simulink model "sampleModel2072_pp"  (R2021a)
settings: Solver=VariableStepAuto  StartTime=0.0  StopTime=10.0  RelTol=1e-3
undefined symbols (not defined in the file or in its folder): DiscIntNeverNeededParam, magnitude, Newton, Raphson
libraries: simulink x184, pid_lib x33
(part 1 of 5)
settings Model: Creator=user  LastModifiedBy=user

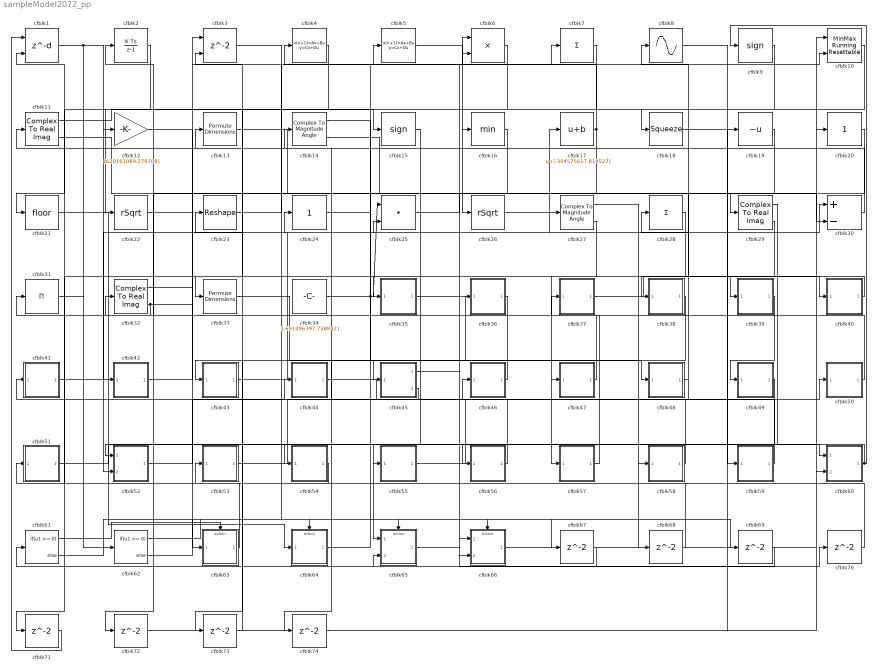
== system sampleModel2072_pp ==
  cfblk1 : Delay  DelayLengthSource=Input port  SampleTime=1
      settings: InputPortMap=u0,p1
  cfblk10 : simulink/Math Operations/MinMax Running Resettable  Function=min  vinit=0.0
  cfblk11 : ComplexToRealImag
  cfblk12 : Gain  Gain=[620161089.279708]
  cfblk13 : PermuteDimensions
  cfblk14 : ComplexToMagnitudeAngle
  cfblk15 : Signum
  cfblk16 : MinMax
  cfblk17 : Bias  Bias=[-304575617.814527]
  cfblk18 : Squeeze
  cfblk19 : UnaryMinus
  cfblk2 : DiscreteIntegrator  ICPrevOutput=DiscIntNeverNeededParam  ICPrevScaledInput=DiscIntNeverNeededParam
  cfblk20 : simulink/Math Operations/Slider Gain  gain=1  low=0  high=2
  cfblk21 : Rounding
  cfblk22 : Sqrt  Operator=rSqrt  AlgorithmType=Newton-Raphson  SaturateOnIntegerOverflow=on
  cfblk23 : Reshape
  cfblk24 : simulink/Math Operations/Slider Gain  gain=1  low=0  high=2
  cfblk25 : DotProduct  InputSameDT=on  OutDataTypeStr=Inherit: Inherit via internal rule
  cfblk26 : Sqrt  Operator=rSqrt  AlgorithmType=Newton-Raphson  SaturateOnIntegerOverflow=on
  cfblk27 : ComplexToMagnitudeAngle
  cfblk28 : Sum  Inputs=+
  cfblk29 : ComplexToRealImag
  cfblk3 : Delay  ShowEnablePort=on  SampleTime=1
      settings: InputPortMap=u0,e6
  cfblk30 : Sum  Inputs=+-
  cfblk31 : Product  Inputs=*
  cfblk32 : ComplexToRealImag
  cfblk33 : PermuteDimensions
  cfblk34 : Constant  Value=[-691496397.738842]  SampleTime=1
  cfblk35 : Subsystem
  cfblk36 : Subsystem
  cfblk37 : Subsystem
  cfblk38 : Subsystem
  cfblk39 : Subsystem
  cfblk4 : DiscreteStateSpace
  cfblk40 : Subsystem
  cfblk41 : Subsystem
  cfblk42 : Subsystem
  cfblk43 : Subsystem
  cfblk44 : Subsystem
  cfblk45 : Subsystem
  cfblk46 : Subsystem
  cfblk47 : Subsystem
  cfblk48 : Subsystem
  cfblk49 : Subsystem
  cfblk5 : DiscreteStateSpace
  cfblk50 : Subsystem
  cfblk51 : Subsystem
  cfblk52 : Subsystem
  cfblk53 : Subsystem
  cfblk54 : Subsystem
  cfblk55 : Subsystem
  cfblk56 : Subsystem
  cfblk57 : Subsystem
  cfblk58 : Subsystem
  cfblk59 : Subsystem
  cfblk6 : Product  Inputs=**
  cfblk60 : Subsystem
  cfblk61 : If  IfExpression=u1 >= 0  SampleTime=1
  cfblk62 : If  IfExpression=u1 >= 0  SampleTime=1
  cfblk63 : Subsystem  TreatAsAtomicUnit=on
  cfblk64 : Subsystem  TreatAsAtomicUnit=on
  cfblk65 : Subsystem  TreatAsAtomicUnit=on
  cfblk66 : Subsystem  TreatAsAtomicUnit=on
  cfblk{67..74} (8 alike) : Delay  SampleTime=1
  cfblk7 : Sum  Inputs=+
  cfblk8 : Sin  TimeSource=Use external signal  SampleTime=0
  cfblk9 : Signum
  wires:
  cfblk10/1 -> cfblk18/1
  cfblk51/1(cfblk2) -> cfblk60/1(cfblk1)
  cfblk35/1(cfblk2) -> cfblk48/1(cfblk1)
  cfblk21/1 -> cfblk64/1(cfblk1)
  cfblk54/1(cfblk2) -> cfblk53/1(cfblk1)
  cfblk34/1 -> cfblk25/1, cfblk7/1
  cfblk4/1 -> cfblk33/1
  cfblk26/1 -> cfblk27/1
  cfblk60/1(cfblk2) -> cfblk9/1, cfblk56/1(cfblk1)
  cfblk39/1(cfblk2) -> cfblk49/1(cfblk1)
  cfblk8/1 -> cfblk59/1(cfblk1)
  cfblk2/1 -> cfblk22/1
  cfblk31/1 -> cfblk42/1(cfblk1)
  cfblk44/1(cfblk2) -> cfblk28/1
  cfblk56/1(cfblk2) -> cfblk23/1
  cfblk66/1(cfblk2) -> cfblk20/1
  cfblk29/1 -> cfblk52/1(cfblk1)
  cfblk30/1 -> cfblk11/1
  cfblk53/1(cfblk2) -> cfblk50/1(cfblk1)
  cfblk50/1(cfblk2) -> cfblk2/1
  cfblk24/1 -> cfblk6/1
  cfblk15/1 -> cfblk35/1(cfblk1)
  cfblk47/1(cfblk2) -> cfblk32/1
  cfblk49/1(cfblk2) -> cfblk65/1(cfblk1)
  cfblk40/1(cfblk2) -> cfblk39/1(cfblk1)
  cfblk9/1 -> cfblk26/1
  cfblk29/2 -> cfblk57/1(cfblk1)
  cfblk41/1(cfblk2) -> cfblk24/1
  cfblk59/1(cfblk2) -> cfblk46/1(cfblk1)
  cfblk46/1(cfblk2) -> cfblk43/1(cfblk1)
  cfblk32/1 -> cfblk3/1
  cfblk5/1 -> cfblk16/1
  cfblk48/1(cfblk2) -> cfblk8/1
  cfblk32/2 -> cfblk25/2, cfblk31/1
  cfblk13/1 -> cfblk36/1(cfblk1)
  cfblk43/1(cfblk2) -> cfblk17/1
  cfblk1/1 -> cfblk12/1, cfblk62/1
  cfblk64/1(cfblk2) -> cfblk30/1
  cfblk7/1 -> cfblk21/1
  cfblk37/1(cfblk2) -> cfblk40/1(cfblk1)
  cfblk19/1 -> cfblk38/1(cfblk1)
  cfblk23/1 -> cfblk5/1
  cfblk17/1 -> cfblk4/1, cfblk66/2(cfblk13)
  cfblk42/1(cfblk2) -> cfblk6/2
  cfblk20/1 -> cfblk45/1(cfblk1)
  cfblk55/1(cfblk2) -> cfblk10/1
  cfblk25/1 -> cfblk10/2
  cfblk11/1 -> cfblk15/1
  cfblk14/1 -> cfblk47/1(cfblk1)
  cfblk58/1(cfblk2) -> cfblk14/1
  cfblk14/2 -> cfblk29/1
  cfblk18/1 -> cfblk30/2
  cfblk6/1 -> cfblk52/2(cfblk16)
  cfblk52/1(cfblk2) -> cfblk44/1(cfblk1)
  cfblk12/1 -> cfblk54/1(cfblk1)
  cfblk57/1(cfblk2) -> cfblk37/1(cfblk1)
  cfblk22/1 -> cfblk63/1(cfblk1)
  cfblk11/2 -> cfblk66/1(cfblk1)
  cfblk27/1 -> cfblk58/1(cfblk1)
  cfblk63/1(cfblk2) -> cfblk51/1(cfblk1)
  cfblk27/2 -> cfblk55/1(cfblk1)
  cfblk45/2(cfblk14) -> cfblk41/1(cfblk1)
  cfblk61/1 -> cfblk63/Action
  cfblk61/2 -> cfblk64/Action
  cfblk62/1 -> cfblk65/Action
  cfblk62/2 -> cfblk66/Action
  cfblk3/1 -> cfblk67/1
  cfblk67/1 -> cfblk61/1
  cfblk33/1 -> cfblk68/1
  cfblk68/1 -> cfblk3/2
  cfblk45/1(cfblk2) -> cfblk69/1
  cfblk69/1 -> cfblk65/2(cfblk9)
  cfblk65/1(cfblk2) -> cfblk70/1
  cfblk70/1 -> cfblk1/2
  cfblk28/1 -> cfblk71/1
  cfblk71/1 -> cfblk1/1
  cfblk16/1 -> cfblk72/1
  cfblk72/1 -> cfblk60/2(cfblk8)
  cfblk36/1(cfblk2) -> cfblk73/1
  cfblk73/1 -> cfblk13/1
  cfblk38/1(cfblk2) -> cfblk74/1
  cfblk74/1 -> cfblk19/1

== system sampleModel2072_pp/cfblk35 ==
  cfblk1 : Inport
  cfblk3 : DiscreteStateSpace
  cfblk4 : Sqrt  SaturateOnIntegerOverflow=on
  cfblk5 : simulink/Math Operations/Slider Gain  gain=1  low=0  high=2
  cfblk6 : Subsystem
  cfblk7 : Subsystem
  cfblk8 : Delay  SampleTime=1
  cfblk2 : Outport
  wires:
  cfblk1/1 -> cfblk7/1(cfblk1)
  cfblk5/1 -> cfblk2/1
  cfblk3/1 -> cfblk4/1
  cfblk7/1(cfblk2) -> cfblk6/1(cfblk1)
  cfblk6/1(cfblk2) -> cfblk5/1
  cfblk4/1 -> cfblk8/1
  cfblk8/1 -> cfblk3/1

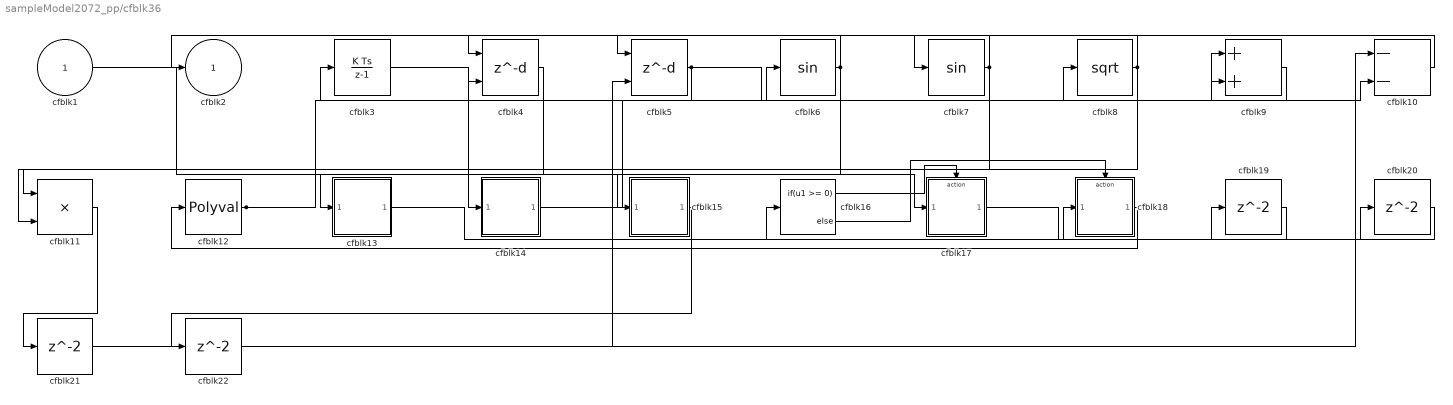
== system sampleModel2072_pp/cfblk36 ==
  cfblk1 : Inport
  cfblk10 : Sum  Inputs=--
  cfblk11 : Product
  cfblk12 : Polyval  Coefs=[ +2.081618890e-019, -1.441693666e-014, +4.719686976e-010, -8.536869453e-006, +1.621573104e-001, -8.087801117e+001 ]
  cfblk13 : Subsystem
  cfblk14 : Subsystem
  cfblk15 : Subsystem
  cfblk16 : If  IfExpression=u1 >= 0  SampleTime=1
  cfblk17 : Subsystem  TreatAsAtomicUnit=on
  cfblk18 : Subsystem  TreatAsAtomicUnit=on
  cfblk{19..22} (4 alike) : Delay  SampleTime=1
  cfblk3 : DiscreteIntegrator  ICPrevOutput=DiscIntNeverNeededParam  ICPrevScaledInput=DiscIntNeverNeededParam
  cfblk4 : Delay  DelayLengthSource=Input port  SampleTime=1
      settings: InputPortMap=u0,p1
  cfblk5 : Delay  DelayLengthSource=Input port  SampleTime=1
      settings: InputPortMap=u0,p1
  cfblk6 : Trigonometry
  cfblk7 : Trigonometry
  cfblk8 : Sqrt  SaturateOnIntegerOverflow=on
  cfblk9 : Sum
  cfblk2 : Outport
  wires:
  cfblk10/1 -> cfblk5/1
  cfblk9/1 -> cfblk6/1
  cfblk5/1 -> cfblk3/1, cfblk9/2
  cfblk7/1 -> cfblk4/1, cfblk11/2
  cfblk1/1 -> cfblk17/1(cfblk1)
  cfblk14/1(cfblk2) -> cfblk8/1
  cfblk8/1 -> cfblk7/1, cfblk11/1
  cfblk3/1 -> cfblk14/1(cfblk1)
  cfblk4/1 -> cfblk13/1(cfblk1)
  cfblk6/1 -> cfblk2/1, cfblk4/2, cfblk15/1(cfblk1)
  cfblk18/1(cfblk2) -> cfblk12/1
  cfblk12/1 -> cfblk10/2, cfblk9/1
  cfblk16/1 -> cfblk17/Action
  cfblk16/2 -> cfblk18/Action
  cfblk17/1(cfblk2) -> cfblk19/1
  cfblk19/1 -> cfblk16/1
  cfblk13/1(cfblk2) -> cfblk20/1
  cfblk20/1 -> cfblk18/1(cfblk1)
  cfblk11/1 -> cfblk21/1
  cfblk21/1 -> cfblk5/2
  cfblk15/1(cfblk2) -> cfblk22/1
  cfblk22/1 -> cfblk10/1

== system sampleModel2072_pp/cfblk37 ==
  cfblk1 : Inport
  cfblk10 : Subsystem
  cfblk11 : Subsystem
  cfblk12 : Delay  SampleTime=1
  cfblk13 : Delay  SampleTime=1
  cfblk3 : pid_lib/PID Controller (2DOF)  Controller=PID  Form=Parallel  TimeDomain=Discrete-time  UseExternalTs=off  SampleTime=1  IntegratorMethod=Forward Euler  FilterMethod=Forward Euler  ControllerParametersSource=internal  P=1  I=1  D=0  UseFilter=on  N=100  b=1  c=1  TunerSelectOption=Transfer Function Based (PID Tuner App)  InitialConditionSource=internal  InitialConditionForIntegrator=0  InitialConditionForFilter=0  DifferentiatorICPrevScaledInput=0  ExternalReset=none  TrackingMode=off  Kt=1  LimitOutput=off  SatLimitsSource=internal  UpperSaturationLimit=inf  LowerSaturationLimit=-inf  LinearizeAsGain=off  AntiWindupMode=none  Kb=1  POutMin=[]  POutMax=[]  IOutMin=[]  IOutMax=[]  DOutMin=[]  DOutMax=[]  NOutMin=[]  NOutMax=[]  bOutMin=[]  bOutMax=[]  cOutMin=[]  cOutMax=[]  SumOutMin=[]  SumOutMax=[]  SaturationOutMin=[]  SaturationOutMax=[]  PParamMin=[]  PParamMax=[]  IParamMin=[]  IParamMax=[]  DParamMin=[]  DParamMax=[]  NParamMin=[]  NParamMax=[]  bParamMin=[]  bParamMax=[]  cParamMin=[]  cParamMax=[]  KbParamMin=[]  KbParamMax=[]  KtParamMin=[]  KtParamMax=[]  KbOutMin=[]  KbOutMax=[]  KtOutMin=[]  KtOutMax=[]  IntegratorOutMin=[]  IntegratorOutMax=[]  FilterOutMin=[]  FilterOutMax=[]  SumI1OutMin=[]  SumI1OutMax=[]  SumI2OutMin=[]  SumI2OutMax=[]  SumI3OutMin=[]  SumI3OutMax=[]  SumI4OutMin=[]  SumI4OutMax=[]  SumDOutMin=[]  SumDOutMax=[]  Sum1OutMin=[]  Sum1OutMax=[]  Sum2OutMin=[]  Sum2OutMax=[]  Sum3OutMin=[]  Sum3OutMax=[]  DifferentiatorOutMin=[]  DifferentiatorOutMax=[]  FilterDiffOutCoefMin=[]  FilterDiffOutCoefMax=[]  ReciprocalOutMin=[]  ReciprocalOutMax=[]  SumDenOutMin=[]  SumDenOutMax=[]  SumNumOutMin=[]  SumNumOutMax=[]  DivideOutMin=[]  DivideOutMax=[]  UdiffTsProdOutMin=[]  UdiffTsProdOutMax=[]  NTsProdOutMin=[]  NTsProdOutMax=[]  UintegralTsProdOutMin=[]  UintegralTsProdOutMax=[]  UngainTsProdOutMin=[]  UngainTsProdOutMax=[]  IntegratorContinuousStateAttributes=''  IntegratorStateMustResolveToSignalObject=off  IntegratorRTWStateStorageClass=Auto  FilterContinuousStateAttributes=''  FilterStateMustResolveToSignalObject=off  FilterRTWStateStorageClass=Auto  ParallelPVariant=InternalParameters  IdealPVariant=Disabled  IVariant=InternalParameters  DVariant=InternalParameters  bVariant=InternalParameters  cVariant=InternalParameters  IntegratorVariant=Discrete  SatVariant=Disabled  AWVariant=Passthrough  PCopyVariant=Disabled  TRVariant=Disabled  FdbkBlocksVariant=Forward  IdealPFdbkVariant=Disabled  SatFdbkVariant=Disabled  DerivativeFilterVariant=ForwardEulerFilter  NVariant=InternalParameters  NCopyVariant=Disabled  FilterICVariant=InternalICsFilter  IntegratorICVariant=InternalICs  ExternalResetVariant=Disabled  TRSumVariant=Passthrough  SumFdbkVariant=Disabled  SumVariant=Sum_PID  TsampFilterVariant=InternalTs  TsampNgainVariant=Passthrough  TsampIntegralVariant=Passthrough  ExternalSaturationOutDataTypeStr=Inherit: Same as second input
      settings: SourceProductBaseCode=SL
  cfblk4 : simulink/Discrete/Transfer Fcn Lead or Lag  PoleZ=0.95  ZeroZ=0.75  ICPrevOutput=0.0  ICPrevInput=0.0  DoSatur=off
      settings: SourceProductBaseCode=SL
  cfblk5 : MinMax  Inputs=2
  cfblk6 : Trigonometry
  cfblk7 : Subsystem
  cfblk8 : Subsystem
  cfblk9 : Subsystem
  cfblk2 : Outport
  wires:
  cfblk1/1 -> cfblk10/1(cfblk1)
  cfblk5/1 -> cfblk4/1
  cfblk10/1(cfblk2) -> cfblk7/1(cfblk1)
  cfblk7/1(cfblk2) -> cfblk8/1(cfblk1)
  cfblk8/1(cfblk2) -> cfblk6/1
  cfblk3/1 -> cfblk2/1, cfblk9/1(cfblk1), cfblk5/2
  cfblk6/1 -> cfblk3/2, cfblk11/1(cfblk1)
  cfblk11/1(cfblk2) -> cfblk5/1
  cfblk9/1(cfblk2) -> cfblk12/1
  cfblk12/1 -> cfblk10/2(cfblk8)
  cfblk4/1 -> cfblk13/1
  cfblk13/1 -> cfblk3/1

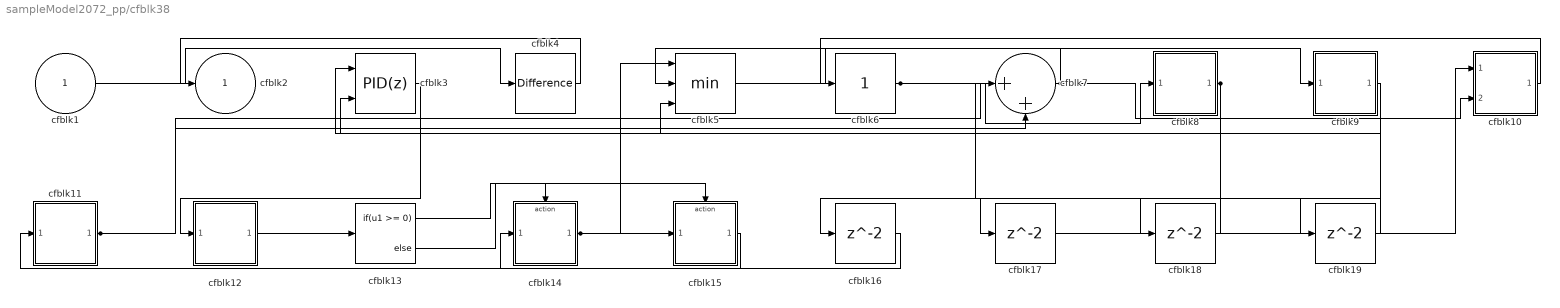
== system sampleModel2072_pp/cfblk38 ==
  cfblk1 : Inport
  cfblk10 : Subsystem
  cfblk11 : Subsystem
  cfblk12 : Subsystem
  cfblk13 : If  IfExpression=u1 >= 0  SampleTime=1
  cfblk14 : Subsystem  TreatAsAtomicUnit=on
  cfblk15 : Subsystem  TreatAsAtomicUnit=on
  cfblk{16..19} (4 alike) : Delay  SampleTime=1
  cfblk3 : pid_lib/PID Controller (2DOF)  Controller=PID  Form=Parallel  TimeDomain=Discrete-time  UseExternalTs=off  SampleTime=1  IntegratorMethod=Forward Euler  FilterMethod=Forward Euler  ControllerParametersSource=internal  P=1  I=1  D=0  UseFilter=on  N=100  b=1  c=1  TunerSelectOption=Transfer Function Based (PID Tuner App)  InitialConditionSource=internal  InitialConditionForIntegrator=0  InitialConditionForFilter=0  DifferentiatorICPrevScaledInput=0  ExternalReset=none  TrackingMode=off  Kt=1  LimitOutput=off  SatLimitsSource=internal  UpperSaturationLimit=inf  LowerSaturationLimit=-inf  LinearizeAsGain=off  AntiWindupMode=none  Kb=1  POutMin=[]  POutMax=[]  IOutMin=[]  IOutMax=[]  DOutMin=[]  DOutMax=[]  NOutMin=[]  NOutMax=[]  bOutMin=[]  bOutMax=[]  cOutMin=[]  cOutMax=[]  SumOutMin=[]  SumOutMax=[]  SaturationOutMin=[]  SaturationOutMax=[]  PParamMin=[]  PParamMax=[]  IParamMin=[]  IParamMax=[]  DParamMin=[]  DParamMax=[]  NParamMin=[]  NParamMax=[]  bParamMin=[]  bParamMax=[]  cParamMin=[]  cParamMax=[]  KbParamMin=[]  KbParamMax=[]  KtParamMin=[]  KtParamMax=[]  KbOutMin=[]  KbOutMax=[]  KtOutMin=[]  KtOutMax=[]  IntegratorOutMin=[]  IntegratorOutMax=[]  FilterOutMin=[]  FilterOutMax=[]  SumI1OutMin=[]  SumI1OutMax=[]  SumI2OutMin=[]  SumI2OutMax=[]  SumI3OutMin=[]  SumI3OutMax=[]  SumI4OutMin=[]  SumI4OutMax=[]  SumDOutMin=[]  SumDOutMax=[]  Sum1OutMin=[]  Sum1OutMax=[]  Sum2OutMin=[]  Sum2OutMax=[]  Sum3OutMin=[]  Sum3OutMax=[]  DifferentiatorOutMin=[]  DifferentiatorOutMax=[]  FilterDiffOutCoefMin=[]  FilterDiffOutCoefMax=[]  ReciprocalOutMin=[]  ReciprocalOutMax=[]  SumDenOutMin=[]  SumDenOutMax=[]  SumNumOutMin=[]  SumNumOutMax=[]  DivideOutMin=[]  DivideOutMax=[]  UdiffTsProdOutMin=[]  UdiffTsProdOutMax=[]  NTsProdOutMin=[]  NTsProdOutMax=[]  UintegralTsProdOutMin=[]  UintegralTsProdOutMax=[]  UngainTsProdOutMin=[]  UngainTsProdOutMax=[]  IntegratorContinuousStateAttributes=''  IntegratorStateMustResolveToSignalObject=off  IntegratorRTWStateStorageClass=Auto  FilterContinuousStateAttributes=''  FilterStateMustResolveToSignalObject=off  FilterRTWStateStorageClass=Auto  ParallelPVariant=InternalParameters  IdealPVariant=Disabled  IVariant=InternalParameters  DVariant=InternalParameters  bVariant=InternalParameters  cVariant=InternalParameters  IntegratorVariant=Discrete  SatVariant=Disabled  AWVariant=Passthrough  PCopyVariant=Disabled  TRVariant=Disabled  FdbkBlocksVariant=Forward  IdealPFdbkVariant=Disabled  SatFdbkVariant=Disabled  DerivativeFilterVariant=ForwardEulerFilter  NVariant=InternalParameters  NCopyVariant=Disabled  FilterICVariant=InternalICsFilter  IntegratorICVariant=InternalICs  ExternalResetVariant=Disabled  TRSumVariant=Passthrough  SumFdbkVariant=Disabled  SumVariant=Sum_PID  TsampFilterVariant=InternalTs  TsampNgainVariant=Passthrough  TsampIntegralVariant=Passthrough  ExternalSaturationOutDataTypeStr=Inherit: Same as second input
      settings: SourceProductBaseCode=SL
  cfblk4 : simulink/Discrete/Difference  ICPrevInput=0.0  OutMin=[]  OutMax=[]  OutDataTypeStr=Inherit: Inherit via back propagation  OutDataType=fixdt(1, 16)  OutScaling=2^-10  DoSatur=off
  cfblk5 : MinMax  Inputs=3
  cfblk6 : simulink/Math Operations/Slider Gain  gain=1  low=0  high=2
  cfblk7 : Sum  Inputs=|++
  cfblk8 : Subsystem
  cfblk9 : Subsystem
  cfblk2 : Outport
  wires:
  cfblk8/1(cfblk2) -> cfblk5/3, cfblk16/1
  cfblk5/1 -> cfblk9/1(cfblk1)
  cfblk3/1 -> cfblk12/1(cfblk1)
  cfblk6/1 -> cfblk8/1(cfblk1), cfblk18/1, cfblk19/1
  cfblk15/1(cfblk2) -> cfblk11/1(cfblk1)
  cfblk14/1(cfblk2) -> cfblk15/1(cfblk1), cfblk5/1
  cfblk1/1 -> cfblk4/1
  cfblk4/1 -> cfblk2/1
  cfblk10/1(cfblk2) -> cfblk6/1
  cfblk12/1(cfblk2) -> cfblk13/1
  cfblk11/1(cfblk2) -> cfblk7/1, cfblk7/2
  cfblk7/1 -> cfblk10/2(cfblk17), cfblk5/2
  cfblk13/1 -> cfblk14/Action
  cfblk13/2 -> cfblk15/Action
  cfblk16/1 -> cfblk14/1(cfblk1)
  cfblk9/1(cfblk2) -> cfblk17/1
  cfblk17/1 -> cfblk10/1(cfblk1)
  cfblk18/1 -> cfblk3/1
  cfblk19/1 -> cfblk3/2

== system sampleModel2072_pp/cfblk39 ==
  cfblk1 : Inport
  cfblk3 : DiscreteFilter  SampleTime=1
  cfblk4 : Sum  Inputs=+-
  cfblk5 : Sum  Inputs=+
  cfblk6 : Subsystem
  cfblk7 : Subsystem
  cfblk8 : Subsystem
  cfblk2 : Outport
  wires:
  cfblk1/1 -> cfblk3/1
  cfblk3/1 -> cfblk6/1(cfblk1)
  cfblk4/1 -> cfblk2/1
  cfblk8/1(cfblk2) -> cfblk5/1
  cfblk6/1(cfblk2) -> cfblk4/1, cfblk7/1(cfblk1)
  cfblk5/1 -> cfblk4/2
  cfblk7/1(cfblk2) -> cfblk8/1(cfblk1)

== system sampleModel2072_pp/cfblk40 ==
  cfblk1 : Inport
  cfblk10 : Subsystem
  cfblk11 : Subsystem
  cfblk12 : Subsystem
  cfblk13 : Delay  SampleTime=1
  cfblk14 : Delay  SampleTime=1
  cfblk3 : simulink/Discrete/Tapped Delay  vinit=0.0  samptime=-1  NumDelays=1  DelayOrder=Oldest  includeCurrent=off
  cfblk4 : Delay  DelayLengthSource=Input port  SampleTime=1
      settings: InputPortMap=u0,p1
  cfblk5 : DiscreteFilter  SampleTime=1
  cfblk6 : simulink/Discrete/Transfer Fcn Real Zero  ZeroZ=0.75  ICPrevInput=0.0  DoSatur=off
      settings: SourceProductBaseCode=SL
  cfblk7 : Squeeze
  cfblk8 : ComplexToRealImag
  cfblk9 : ComplexToRealImag
  cfblk2 : Outport
  wires:
  cfblk10/1(cfblk2) -> cfblk4/1
  cfblk11/1(cfblk2) -> cfblk2/1
  cfblk3/1 -> cfblk11/1(cfblk1)
  cfblk7/1 -> cfblk9/1
  cfblk8/1 -> cfblk10/1(cfblk1)
  cfblk9/1 -> cfblk8/1
  cfblk4/1 -> cfblk6/1
  cfblk1/1 -> cfblk5/1
  cfblk9/2 -> cfblk3/1
  cfblk8/2 -> cfblk12/1(cfblk1)
  cfblk5/1 -> cfblk10/2(cfblk8)
  cfblk6/1 -> cfblk13/1
  cfblk13/1 -> cfblk4/2
  cfblk12/1(cfblk2) -> cfblk14/1
  cfblk14/1 -> cfblk7/1

== system sampleModel2072_pp/cfblk41 ==
  cfblk1 : Inport
  cfblk10 : Subsystem
  cfblk11 : Subsystem
  cfblk12 : Delay  SampleTime=1
  cfblk13 : Delay  SampleTime=1
  cfblk3 : DiscreteIntegrator  ICPrevOutput=DiscIntNeverNeededParam  ICPrevScaledInput=DiscIntNeverNeededParam
  cfblk4 : MinMax  Inputs=3
  cfblk5 : simulink/Math Operations/Slider Gain  gain=1  low=0  high=2
  cfblk6 : simulink/Math Operations/Slider Gain  gain=1  low=0  high=2
  cfblk7 : Subsystem
  cfblk8 : Subsystem
  cfblk9 : Subsystem
  cfblk2 : Outport
  wires:
  cfblk4/1 -> cfblk10/1(cfblk1)
  cfblk7/1(cfblk2) -> cfblk11/1(cfblk1), cfblk12/1
  cfblk10/1(cfblk2) -> cfblk7/1(cfblk1)
  cfblk1/1 -> cfblk8/1(cfblk1)
  cfblk9/1(cfblk2) -> cfblk5/1
  cfblk11/1(cfblk2) -> cfblk2/1
  cfblk5/1 -> cfblk4/1
  cfblk8/1(cfblk2) -> cfblk9/1(cfblk1), cfblk4/3
  cfblk3/1 -> cfblk6/1
  cfblk12/1 -> cfblk4/2
  cfblk6/1 -> cfblk13/1
  cfblk13/1 -> cfblk3/1

== system sampleModel2072_pp/cfblk42 ==
  cfblk1 : Inport
  cfblk3 : Abs
  cfblk4 : Subsystem
  cfblk5 : Subsystem
  cfblk6 : Subsystem
  cfblk7 : Subsystem
  cfblk8 : Delay  SampleTime=1
  cfblk2 : Outport
  wires:
  cfblk4/1(cfblk2) -> cfblk7/1(cfblk1)
  cfblk6/1(cfblk2) -> cfblk4/1(cfblk1)
  cfblk1/1 -> cfblk2/1
  cfblk7/1(cfblk2) -> cfblk5/1(cfblk1)
  cfblk3/1 -> cfblk6/1(cfblk1)
  cfblk5/1(cfblk2) -> cfblk8/1
  cfblk8/1 -> cfblk3/1

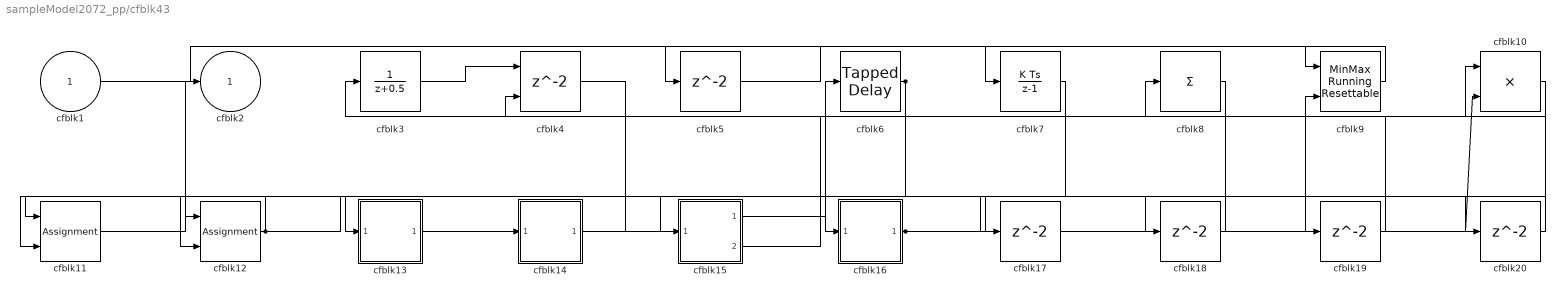
== system sampleModel2072_pp/cfblk43 ==
  cfblk1 : Inport
  cfblk10 : Product
  cfblk11 : Assignment  DiagnosticForDimensions=Warning  IndexOptions=Index vector (dialog)  Indices=1  OutputSizes=1
  cfblk12 : Assignment  DiagnosticForDimensions=Warning  IndexOptions=Index vector (dialog)  Indices=1  OutputSizes=1
  cfblk13 : Subsystem
  cfblk14 : Subsystem
  cfblk15 : Subsystem
  cfblk16 : Subsystem
  cfblk{5,17..20} (5 alike) : Delay  SampleTime=1
  cfblk3 : DiscreteTransferFcn  SampleTime=1
  cfblk4 : Delay  ShowEnablePort=on  SampleTime=1
      settings: InputPortMap=u0,e6
  cfblk6 : simulink/Discrete/Tapped Delay  vinit=0.0  samptime=-1  NumDelays=1  DelayOrder=Oldest  includeCurrent=off
  cfblk7 : DiscreteIntegrator  ICPrevOutput=DiscIntNeverNeededParam  ICPrevScaledInput=DiscIntNeverNeededParam
  cfblk8 : Sum  Inputs=+
  cfblk9 : simulink/Math Operations/MinMax Running Resettable  Function=min  vinit=0.0
  cfblk2 : Outport
  wires:
  cfblk1/1 -> cfblk9/1
  cfblk3/1 -> cfblk4/1
  cfblk4/1 -> cfblk15/1(cfblk1)
  cfblk14/1(cfblk2) -> cfblk16/1(cfblk1)
  cfblk15/1(cfblk2) -> cfblk6/1
  cfblk5/1 -> cfblk7/1
  cfblk12/1 -> cfblk11/1, cfblk18/1
  cfblk8/1 -> cfblk13/1(cfblk1)
  cfblk13/1(cfblk2) -> cfblk14/1(cfblk1)
  cfblk6/1 -> cfblk11/2, cfblk12/1, cfblk12/2
  cfblk9/1 -> cfblk5/1
  cfblk15/2(cfblk10) -> cfblk10/1
  cfblk16/1(cfblk2) -> cfblk10/2, cfblk20/1
  cfblk11/1 -> cfblk2/1
  cfblk7/1 -> cfblk17/1
  cfblk17/1 -> cfblk9/2
  cfblk18/1 -> cfblk4/2
  cfblk10/1 -> cfblk19/1
  cfblk19/1 -> cfblk3/1
  cfblk20/1 -> cfblk8/1

== system sampleModel2072_pp/cfblk44 ==
  cfblk1 : Inport
  cfblk10 : UnaryMinus
  cfblk11 : Subsystem
  cfblk12 : Subsystem
  cfblk13 : If  IfExpression=u1 >= 0  SampleTime=1
  cfblk14 : Subsystem  TreatAsAtomicUnit=on
  cfblk15 : Subsystem  TreatAsAtomicUnit=on
  cfblk16 : Delay  SampleTime=1
  cfblk17 : Delay  SampleTime=1
  cfblk3 : Sum  Inputs=+
  cfblk4 : Assignment  DiagnosticForDimensions=Warning  IndexOptions=Index vector (dialog)  Indices=1  OutputSizes=1
  cfblk5 : Sum  Inputs=+-
  cfblk6 : Assignment  DiagnosticForDimensions=Warning  IndexOptions=Index vector (dialog)  Indices=1  OutputSizes=1
  cfblk7 : Sqrt  Operator=rSqrt  AlgorithmType=Newton-Raphson  SaturateOnIntegerOverflow=on
  cfblk8 : Sqrt  Operator=rSqrt  AlgorithmType=Newton-Raphson  SaturateOnIntegerOverflow=on
  cfblk9 : Squeeze
  cfblk2 : Outport
  wires:
  cfblk7/1 -> cfblk11/1(cfblk1)
  cfblk1/1 -> cfblk13/1
  cfblk12/1(cfblk2) -> cfblk10/1
  cfblk11/1(cfblk2) -> cfblk5/1, cfblk17/1
  cfblk9/1 -> cfblk3/1
  cfblk4/1 -> cfblk7/1
  cfblk14/1(cfblk2) -> cfblk12/1(cfblk1), cfblk4/2, cfblk15/1(cfblk1)
  cfblk10/1 -> cfblk6/1
  cfblk5/1 -> cfblk8/1, cfblk16/1
  cfblk3/1 -> cfblk5/2
  cfblk6/1 -> cfblk9/1
  cfblk8/1 -> cfblk2/1
  cfblk15/1(cfblk2) -> cfblk6/2
  cfblk13/1 -> cfblk14/Action
  cfblk13/2 -> cfblk15/Action
  cfblk16/1 -> cfblk14/1(cfblk1)
  cfblk17/1 -> cfblk4/1

== system sampleModel2072_pp/cfblk45 ==
  cfblk1 : Inport
  cfblk10 : ComplexToRealImag
  cfblk11 : Trigonometry
  cfblk12 : Subsystem
  cfblk13 : Subsystem
  cfblk15 : Delay  SampleTime=1
  cfblk16 : Delay  SampleTime=1
  cfblk17 : Delay  SampleTime=1
  cfblk3 : DiscreteZeroPole  Poles=[0 0.5]  Gain=1
  cfblk4 : DiscreteFir  SampleTime=1
  cfblk5 : DiscreteStateSpace
  cfblk6 : Bias  Bias=[927380128.816575]
  cfblk7 : Abs
  cfblk8 : Product
  cfblk9 : Assignment  DiagnosticForDimensions=Warning  IndexOptions=Index vector (dialog)  Indices=1  OutputSizes=1
  cfblk2 : Outport
  cfblk14 : Outport  Port=2
  wires:
  cfblk3/1 -> cfblk5/1
  cfblk9/1 -> cfblk7/1, cfblk12/1(cfblk1)
  cfblk11/1 -> cfblk6/1, cfblk17/1
  cfblk5/1 -> cfblk4/1
  cfblk7/1 -> cfblk10/1
  cfblk8/1 -> cfblk13/1(cfblk1)
  cfblk4/1 -> cfblk9/2
  cfblk1/1 -> cfblk8/2
  cfblk6/1 -> cfblk2/1
  cfblk10/2 -> cfblk14/1
  cfblk12/1(cfblk2) -> cfblk11/1
  cfblk13/1(cfblk2) -> cfblk15/1
  cfblk15/1 -> cfblk8/1
  cfblk10/1 -> cfblk16/1
  cfblk16/1 -> cfblk3/1
  cfblk17/1 -> cfblk9/1

== system sampleModel2072_pp/cfblk46 ==
  cfblk1 : Inport
  cfblk10 : Subsystem
  cfblk11 : Subsystem
  cfblk12 : Subsystem
  cfblk13 : Delay  SampleTime=1
  cfblk3 : Gain  Gain=[-231739118.082648]
  cfblk4 : ComplexToRealImag
  cfblk5 : Rounding
  cfblk6 : Polyval  Coefs=[ +2.081618890e-019, -1.441693666e-014, +4.719686976e-010, -8.536869453e-006, +1.621573104e-001, -8.087801117e+001 ]
  cfblk7 : Rounding
  cfblk8 : Sum  Inputs=+
  cfblk9 : Subsystem
  cfblk2 : Outport
  wires:
  cfblk1/1 -> cfblk10/1(cfblk1), cfblk4/1
  cfblk10/1(cfblk2) -> cfblk6/1
  cfblk11/1(cfblk2) -> cfblk12/1(cfblk1)
  cfblk3/1 -> cfblk11/1(cfblk1)
  cfblk8/1 -> cfblk9/1(cfblk1)
  cfblk7/1 -> cfblk8/1
  cfblk6/1 -> cfblk7/1
  cfblk12/1(cfblk2) -> cfblk5/1
  cfblk9/1(cfblk2) -> cfblk2/1
  cfblk5/1 -> cfblk13/1
  cfblk13/1 -> cfblk3/1

== system sampleModel2072_pp/cfblk47 ==
  cfblk1 : Inport
  cfblk10 : Abs
  cfblk11 : DotProduct  InputSameDT=on  OutDataTypeStr=Inherit: Inherit via internal rule
  cfblk12 : Assignment  DiagnosticForDimensions=Warning  IndexOptions=Index vector (dialog)  Indices=1  OutputSizes=1
  cfblk13 : Subsystem
  cfblk14 : Delay  SampleTime=1
  cfblk15 : Delay  SampleTime=1
  cfblk3 : simulink/Discrete/Transfer Fcn Lead or Lag  PoleZ=0.95  ZeroZ=0.75  ICPrevOutput=0.0  ICPrevInput=0.0  DoSatur=off
      settings: SourceProductBaseCode=SL
  cfblk4 : DiscreteIntegrator  ICPrevOutput=DiscIntNeverNeededParam  ICPrevScaledInput=DiscIntNeverNeededParam
  cfblk5 : DiscreteTransferFcn  SampleTime=1
  cfblk6 : DiscreteStateSpace
  cfblk7 : simulink/Discrete/Transfer Fcn Real Zero  ZeroZ=0.75  ICPrevInput=0.0  DoSatur=off
      settings: SourceProductBaseCode=SL
  cfblk8 : simulink/Math Operations/Slider Gain  gain=1  low=0  high=2
  cfblk9 : Sqrt  Operator=rSqrt  AlgorithmType=Newton-Raphson  SaturateOnIntegerOverflow=on
  cfblk2 : Outport
  wires:
  cfblk6/1 -> cfblk12/2
  cfblk11/1 -> cfblk13/1(cfblk1), cfblk2/1
  cfblk12/1 -> cfblk9/1
  cfblk9/1 -> cfblk5/1
  cfblk4/1 -> cfblk6/1
  cfblk1/1 -> cfblk7/1, cfblk4/1
  cfblk8/1 -> cfblk3/1
  cfblk3/1 -> cfblk11/1
  cfblk5/1 -> cfblk10/1
  cfblk7/1 -> cfblk8/1
  cfblk13/1(cfblk2) -> cfblk14/1
  cfblk14/1 -> cfblk11/2
  cfblk10/1 -> cfblk15/1
  cfblk15/1 -> cfblk12/1

== system sampleModel2072_pp/cfblk48 ==
  cfblk1 : Inport
  cfblk3 : Gain  Gain=[318994454.950710]
  cfblk4 : ComplexToRealImag
  cfblk5 : Polyval  Coefs=[ +2.081618890e-019, -1.441693666e-014, +4.719686976e-010, -8.536869453e-006, +1.621573104e-001, -8.087801117e+001 ]
  cfblk6 : Sin  TimeSource=Use external signal  SampleTime=0
  cfblk7 : Sum  Inputs=+-
  cfblk8 : Delay  SampleTime=1
  cfblk2 : Outport
  wires:
  cfblk3/1 -> cfblk6/1
  cfblk5/1 -> cfblk2/1
  cfblk4/1 -> cfblk5/1
  cfblk1/1 -> cfblk4/1
  cfblk7/1 -> cfblk3/1
  cfblk4/2 -> cfblk7/2
  cfblk6/1 -> cfblk8/1
  cfblk8/1 -> cfblk7/1

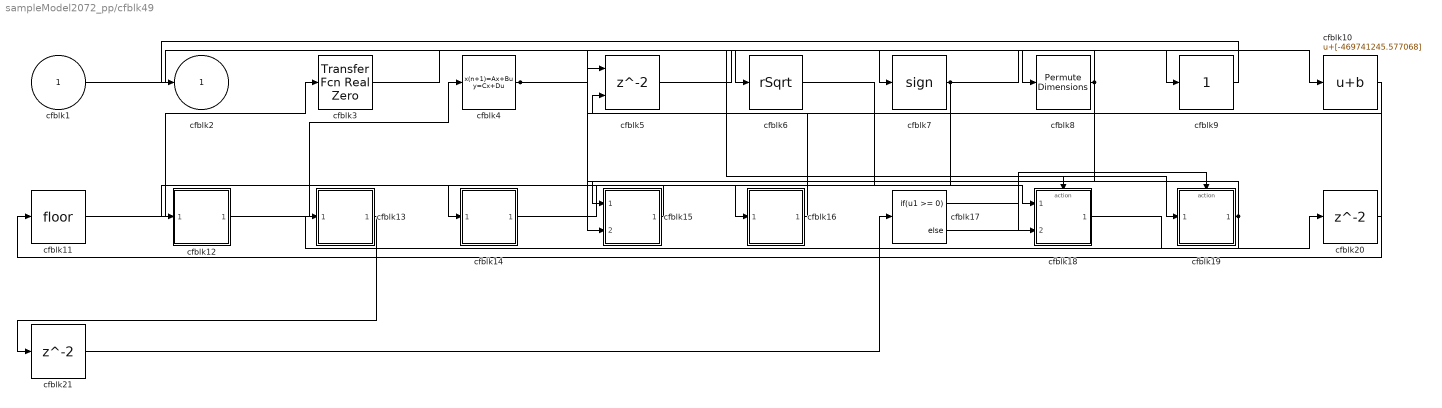
== system sampleModel2072_pp/cfblk49 ==
  cfblk1 : Inport
  cfblk10 : Bias  Bias=[-469741245.577068]
  cfblk11 : Rounding
  cfblk12 : Subsystem
  cfblk13 : Subsystem
  cfblk14 : Subsystem
  cfblk15 : Subsystem
  cfblk16 : Subsystem
  cfblk17 : If  IfExpression=u1 >= 0  SampleTime=1
  cfblk18 : Subsystem  TreatAsAtomicUnit=on
  cfblk19 : Subsystem  TreatAsAtomicUnit=on
  cfblk20 : Delay  SampleTime=1
  cfblk21 : Delay  SampleTime=1
  cfblk3 : simulink/Discrete/Transfer Fcn Real Zero  ZeroZ=0.75  ICPrevInput=0.0  DoSatur=off
      settings: SourceProductBaseCode=SL
  cfblk4 : DiscreteStateSpace
  cfblk5 : Delay  ShowEnablePort=on  SampleTime=1
      settings: InputPortMap=u0,e6
  cfblk6 : Sqrt  Operator=rSqrt  AlgorithmType=Newton-Raphson  SaturateOnIntegerOverflow=on
  cfblk7 : Signum
  cfblk8 : PermuteDimensions
  cfblk9 : simulink/Math Operations/Slider Gain  gain=1  low=0  high=2
  cfblk2 : Outport
  wires:
  cfblk11/1 -> cfblk3/1
  cfblk12/1(cfblk2) -> cfblk4/1
  cfblk19/1(cfblk2) -> cfblk13/1(cfblk1), cfblk15/1(cfblk1)
  cfblk8/1 -> cfblk6/1, cfblk15/2(cfblk11)
  cfblk3/1 -> cfblk19/1(cfblk1)
  cfblk1/1 -> cfblk7/1
  cfblk15/1(cfblk2) -> cfblk12/1(cfblk1)
  cfblk5/1 -> cfblk8/1
  cfblk9/1 -> cfblk2/1
  cfblk10/1 -> cfblk11/1
  cfblk7/1 -> cfblk14/1(cfblk1), cfblk10/1
  cfblk16/1(cfblk2) -> cfblk5/2
  cfblk14/1(cfblk2) -> cfblk16/1(cfblk1)
  cfblk6/1 -> cfblk18/1(cfblk1)
  cfblk4/1 -> cfblk9/1, cfblk18/2(cfblk15)
  cfblk17/1 -> cfblk18/Action
  cfblk17/2 -> cfblk19/Action
  cfblk18/1(cfblk2) -> cfblk20/1
  cfblk20/1 -> cfblk5/1
  cfblk13/1(cfblk2) -> cfblk21/1
  cfblk21/1 -> cfblk17/1

== system sampleModel2072_pp/cfblk50 ==
  cfblk1 : Inport
  cfblk10 : Delay  SampleTime=1
  cfblk3 : simulink/Discrete/Difference  ICPrevInput=0.0  OutMin=[]  OutMax=[]  OutDataTypeStr=Inherit: Inherit via back propagation  OutDataType=fixdt(1, 16)  OutScaling=2^-10  DoSatur=off
  cfblk4 : DiscreteTransferFcn  SampleTime=1
  cfblk5 : DiscreteIntegrator  ICPrevOutput=DiscIntNeverNeededParam  ICPrevScaledInput=DiscIntNeverNeededParam
  cfblk6 : ComplexToRealImag
  cfblk7 : simulink/Math Operations/Slider Gain  gain=1  low=0  high=2
  cfblk8 : Bias  Bias=[-640892454.891327]
  cfblk9 : Assignment  DiagnosticForDimensions=Warning  IndexOptions=Index vector (dialog)  Indices=1  OutputSizes=1
  cfblk2 : Outport
  wires:
  cfblk5/1 -> cfblk7/1
  cfblk7/1 -> cfblk6/1
  cfblk6/1 -> cfblk9/1
  cfblk4/1 -> cfblk5/1
  cfblk6/2 -> cfblk8/1
  cfblk9/1 -> cfblk2/1
  cfblk1/1 -> cfblk3/1
  cfblk3/1 -> cfblk9/2
  cfblk8/1 -> cfblk10/1
  cfblk10/1 -> cfblk4/1

== system sampleModel2072_pp/cfblk51 ==
  cfblk1 : Inport
  cfblk10 : Delay  SampleTime=1
  cfblk3 : simulink/Discrete/Transfer Fcn First Order  PoleZ=0.95  ICPrevOutput=0.0  DoSatur=off
  cfblk4 : simulink/Discrete/Tapped Delay  vinit=0.0  samptime=-1  NumDelays=1  DelayOrder=Oldest  includeCurrent=off
  cfblk5 : Rounding
  cfblk6 : Subsystem
  cfblk7 : Subsystem
  cfblk8 : Subsystem
  cfblk9 : Subsystem
  cfblk2 : Outport
  wires:
  cfblk3/1 -> cfblk7/1(cfblk1)
  cfblk9/1(cfblk2) -> cfblk6/1(cfblk1)
  cfblk5/1 -> cfblk9/1(cfblk1)
  cfblk7/1(cfblk2) -> cfblk8/1(cfblk1)
  cfblk4/1 -> cfblk3/1
  cfblk1/1 -> cfblk4/1
  cfblk8/1(cfblk2) -> cfblk2/1
  cfblk6/1(cfblk2) -> cfblk10/1
  cfblk10/1 -> cfblk5/1

== system sampleModel2072_pp/cfblk52 ==
  cfblk1 : Inport
  cfblk16 : Inport  Port=2
  cfblk10 : Polyval  Coefs=[ +2.081618890e-019, -1.441693666e-014, +4.719686976e-010, -8.536869453e-006, +1.621573104e-001, -8.087801117e+001 ]
  cfblk11 : UnaryMinus
  cfblk12 : Constant  Value=[384477365.169266]  SampleTime=1
  cfblk13 : Subsystem
  cfblk14 : Subsystem
  cfblk15 : Subsystem
  cfblk17 : Delay  SampleTime=1
  cfblk3 : pid_lib/PID Controller (2DOF)  Controller=PID  Form=Parallel  TimeDomain=Discrete-time  UseExternalTs=off  SampleTime=1  IntegratorMethod=Forward Euler  FilterMethod=Forward Euler  ControllerParametersSource=internal  P=1  I=1  D=0  UseFilter=on  N=100  b=1  c=1  TunerSelectOption=Transfer Function Based (PID Tuner App)  InitialConditionSource=internal  InitialConditionForIntegrator=0  InitialConditionForFilter=0  DifferentiatorICPrevScaledInput=0  ExternalReset=none  TrackingMode=off  Kt=1  LimitOutput=off  SatLimitsSource=internal  UpperSaturationLimit=inf  LowerSaturationLimit=-inf  LinearizeAsGain=off  AntiWindupMode=none  Kb=1  POutMin=[]  POutMax=[]  IOutMin=[]  IOutMax=[]  DOutMin=[]  DOutMax=[]  NOutMin=[]  NOutMax=[]  bOutMin=[]  bOutMax=[]  cOutMin=[]  cOutMax=[]  SumOutMin=[]  SumOutMax=[]  SaturationOutMin=[]  SaturationOutMax=[]  PParamMin=[]  PParamMax=[]  IParamMin=[]  IParamMax=[]  DParamMin=[]  DParamMax=[]  NParamMin=[]  NParamMax=[]  bParamMin=[]  bParamMax=[]  cParamMin=[]  cParamMax=[]  KbParamMin=[]  KbParamMax=[]  KtParamMin=[]  KtParamMax=[]  KbOutMin=[]  KbOutMax=[]  KtOutMin=[]  KtOutMax=[]  IntegratorOutMin=[]  IntegratorOutMax=[]  FilterOutMin=[]  FilterOutMax=[]  SumI1OutMin=[]  SumI1OutMax=[]  SumI2OutMin=[]  SumI2OutMax=[]  SumI3OutMin=[]  SumI3OutMax=[]  SumI4OutMin=[]  SumI4OutMax=[]  SumDOutMin=[]  SumDOutMax=[]  Sum1OutMin=[]  Sum1OutMax=[]  Sum2OutMin=[]  Sum2OutMax=[]  Sum3OutMin=[]  Sum3OutMax=[]  DifferentiatorOutMin=[]  DifferentiatorOutMax=[]  FilterDiffOutCoefMin=[]  FilterDiffOutCoefMax=[]  ReciprocalOutMin=[]  ReciprocalOutMax=[]  SumDenOutMin=[]  SumDenOutMax=[]  SumNumOutMin=[]  SumNumOutMax=[]  DivideOutMin=[]  DivideOutMax=[]  UdiffTsProdOutMin=[]  UdiffTsProdOutMax=[]  NTsProdOutMin=[]  NTsProdOutMax=[]  UintegralTsProdOutMin=[]  UintegralTsProdOutMax=[]  UngainTsProdOutMin=[]  UngainTsProdOutMax=[]  IntegratorContinuousStateAttributes=''  IntegratorStateMustResolveToSignalObject=off  IntegratorRTWStateStorageClass=Auto  FilterContinuousStateAttributes=''  FilterStateMustResolveToSignalObject=off  FilterRTWStateStorageClass=Auto  ParallelPVariant=InternalParameters  IdealPVariant=Disabled  IVariant=InternalParameters  DVariant=InternalParameters  bVariant=InternalParameters  cVariant=InternalParameters  IntegratorVariant=Discrete  SatVariant=Disabled  AWVariant=Passthrough  PCopyVariant=Disabled  TRVariant=Disabled  FdbkBlocksVariant=Forward  IdealPFdbkVariant=Disabled  SatFdbkVariant=Disabled  DerivativeFilterVariant=ForwardEulerFilter  NVariant=InternalParameters  NCopyVariant=Disabled  FilterICVariant=InternalICsFilter  IntegratorICVariant=InternalICs  ExternalResetVariant=Disabled  TRSumVariant=Passthrough  SumFdbkVariant=Disabled  SumVariant=Sum_PID  TsampFilterVariant=InternalTs  TsampNgainVariant=Passthrough  TsampIntegralVariant=Passthrough  ExternalSaturationOutDataTypeStr=Inherit: Same as second input
      settings: SourceProductBaseCode=SL
  cfblk4 : DiscreteZeroPole  Poles=[0 0.5]  Gain=1
  cfblk5 : Product  Inputs=**
  cfblk6 : Sum  Inputs=+
  cfblk7 : Squeeze
  cfblk8 : ComplexToRealImag
  cfblk9 : Assignment  DiagnosticForDimensions=Warning  IndexOptions=Index vector (dialog)  Indices=1  OutputSizes=1
  cfblk2 : Outport
  wires:
  cfblk11/1 -> cfblk9/1
  cfblk5/1 -> cfblk8/1
  cfblk4/1 -> cfblk7/1
  cfblk3/1 -> cfblk4/1
  cfblk8/1 -> cfblk2/1
  cfblk16/1 -> cfblk6/1
  cfblk6/1 -> cfblk14/1(cfblk1)
  cfblk7/1 -> cfblk10/1
  cfblk12/1 -> cfblk9/2
  cfblk10/1 -> cfblk15/1(cfblk1)
  cfblk9/1 -> cfblk5/1
  cfblk15/1(cfblk2) -> cfblk11/1
  cfblk8/2 -> cfblk13/1(cfblk1), cfblk17/1
  cfblk14/1(cfblk2) -> cfblk5/2
  cfblk1/1 -> cfblk3/2
  cfblk17/1 -> cfblk3/1

== system sampleModel2072_pp/cfblk53 ==
  cfblk1 : Inport
  cfblk10 : Subsystem
  cfblk11 : Subsystem
  cfblk12 : Delay  SampleTime=1
  cfblk13 : Delay  SampleTime=1
  cfblk3 : simulink/Discrete/Tapped Delay  vinit=0.0  samptime=-1  NumDelays=1  DelayOrder=Oldest  includeCurrent=off
  cfblk4 : Sqrt  Operator=rSqrt  AlgorithmType=Newton-Raphson  SaturateOnIntegerOverflow=on
  cfblk5 : Sum  Inputs=+
  cfblk6 : Rounding
  cfblk7 : Sum
  cfblk8 : Subsystem
  cfblk9 : Subsystem
  cfblk2 : Outport
  wires:
  cfblk11/1(cfblk2) -> cfblk2/1
  cfblk3/1 -> cfblk10/1(cfblk1), cfblk4/1
  cfblk8/1(cfblk2) -> cfblk6/1, cfblk12/1
  cfblk1/1 -> cfblk5/1
  cfblk10/1(cfblk2) -> cfblk9/1(cfblk1)
  cfblk7/1 -> cfblk8/1(cfblk1)
  cfblk9/1(cfblk2) -> cfblk7/1
  cfblk5/1 -> cfblk10/2(cfblk13)
  cfblk6/1 -> cfblk11/1(cfblk1)
  cfblk12/1 -> cfblk7/2
  cfblk4/1 -> cfblk13/1
  cfblk13/1 -> cfblk3/1

== system sampleModel2072_pp/cfblk54 ==
  cfblk1 : Inport
  cfblk10 : Subsystem
  cfblk11 : Subsystem
  cfblk12 : Subsystem
  cfblk13 : Subsystem
  cfblk{3,14..16} (4 alike) : Delay  SampleTime=1
  cfblk4 : DotProduct  InputSameDT=on  OutDataTypeStr=Inherit: Inherit via internal rule
  cfblk5 : simulink/Math Operations/MinMax Running Resettable  Function=min  vinit=0.0
  cfblk6 : Product
  cfblk7 : Sqrt  Operator=rSqrt  AlgorithmType=Newton-Raphson  SaturateOnIntegerOverflow=on
  cfblk8 : Subsystem
  cfblk9 : Subsystem
  cfblk2 : Outport
  wires:
  cfblk10/1(cfblk2) -> cfblk7/1
  cfblk5/1 -> cfblk11/1(cfblk1), cfblk12/1(cfblk1)
  cfblk12/1(cfblk2) -> cfblk13/1(cfblk1)
  cfblk13/1(cfblk2) -> cfblk3/1, cfblk8/1(cfblk1)
  cfblk1/1 -> cfblk2/1
  cfblk11/1(cfblk2) -> cfblk9/1(cfblk1)
  cfblk8/1(cfblk2) -> cfblk15/1, cfblk16/1
  cfblk7/1 -> cfblk4/1
  cfblk6/1 -> cfblk10/1(cfblk1)
  cfblk3/1 -> cfblk6/2
  cfblk9/1(cfblk2) -> cfblk4/2
  cfblk4/1 -> cfblk14/1
  cfblk14/1 -> cfblk6/1
  cfblk15/1 -> cfblk5/1
  cfblk16/1 -> cfblk5/2

== system sampleModel2072_pp/cfblk55 ==
  cfblk1 : Inport
  cfblk10 : Polyval  Coefs=[ +2.081618890e-019, -1.441693666e-014, +4.719686976e-010, -8.536869453e-006, +1.621573104e-001, -8.087801117e+001 ]
  cfblk11 : Subsystem
  cfblk12 : Subsystem
  cfblk13 : Delay  SampleTime=1
  cfblk3 : simulink/Discrete/Transfer Fcn Real Zero  ZeroZ=0.75  ICPrevInput=0.0  DoSatur=off
      settings: SourceProductBaseCode=SL
  cfblk4 : UnitDelay  HasFrameUpgradeWarning=on
  cfblk5 : DiscreteStateSpace
  cfblk6 : simulink/Discrete/Transfer Fcn Real Zero  ZeroZ=0.75  ICPrevInput=0.0  DoSatur=off
      settings: SourceProductBaseCode=SL
  cfblk7 : Assignment  DiagnosticForDimensions=Warning  IndexOptions=Index vector (dialog)  Indices=1  OutputSizes=1
  cfblk8 : Bias  Bias=[-821428964.335241]
  cfblk9 : Sqrt  Operator=rSqrt  AlgorithmType=Newton-Raphson  SaturateOnIntegerOverflow=on
  cfblk2 : Outport
  wires:
  cfblk7/1 -> cfblk10/1
  cfblk8/1 -> cfblk11/1(cfblk1)
  cfblk11/1(cfblk2) -> cfblk6/1, cfblk9/1
  cfblk5/1 -> cfblk2/1
  cfblk9/1 -> cfblk5/1
  cfblk3/1 -> cfblk4/1
  cfblk10/1 -> cfblk12/1(cfblk1)
  cfblk4/1 -> cfblk8/1
  cfblk6/1 -> cfblk7/2
  cfblk1/1 -> cfblk3/1
  cfblk12/1(cfblk2) -> cfblk13/1
  cfblk13/1 -> cfblk7/1

== system sampleModel2072_pp/cfblk56 ==
  cfblk1 : Inport
  cfblk10 : Assignment  DiagnosticForDimensions=Warning  IndexOptions=Index vector (dialog)  Indices=1  OutputSizes=1
  cfblk11 : Squeeze
  cfblk12 : Sqrt  Operator=rSqrt  AlgorithmType=Newton-Raphson  SaturateOnIntegerOverflow=on
  cfblk13 : Subsystem
  cfblk14 : Subsystem
  cfblk15 : Delay  SampleTime=1
  cfblk3 : Delay  SampleTime=1
  cfblk4 : DiscreteFilter  SampleTime=1
  cfblk5 : DiscreteTransferFcn  SampleTime=1
  cfblk6 : Math  Operator=magnitude^2  SaturateOnIntegerOverflow=on
  cfblk7 : Gain  Gain=[113117787.399551]
  cfblk8 : Sqrt  Operator=rSqrt  AlgorithmType=Newton-Raphson  SaturateOnIntegerOverflow=on
  cfblk9 : ComplexToMagnitudeAngle
  cfblk2 : Outport
  wires:
  cfblk10/1 -> cfblk3/1
  cfblk1/1 -> cfblk12/1
  cfblk12/1 -> cfblk5/1
  cfblk11/1 -> cfblk6/1
  cfblk6/1 -> cfblk10/1
  cfblk14/1(cfblk2) -> cfblk11/1
  cfblk3/1 -> cfblk2/1
  cfblk5/1 -> cfblk10/2
  cfblk4/1 -> cfblk8/1
  cfblk9/1 -> cfblk4/1
  cfblk7/1 -> cfblk13/1(cfblk1), cfblk9/1
  cfblk8/1 -> cfblk14/1(cfblk1)
  cfblk13/1(cfblk2) -> cfblk15/1
  cfblk15/1 -> cfblk7/1

== system sampleModel2072_pp/cfblk57 ==
  cfblk1 : Inport
  cfblk10 : Subsystem
  cfblk11 : Subsystem
  cfblk12 : Subsystem
  cfblk13 : Delay  SampleTime=1
  cfblk14 : Delay  SampleTime=1
  cfblk15 : Delay  SampleTime=1
  cfblk3 : DiscreteIntegrator  ICPrevOutput=DiscIntNeverNeededParam  ICPrevScaledInput=DiscIntNeverNeededParam
  cfblk4 : Trigonometry
  cfblk5 : Product
  cfblk6 : Polyval  Coefs=[ +2.081618890e-019, -1.441693666e-014, +4.719686976e-010, -8.536869453e-006, +1.621573104e-001, -8.087801117e+001 ]
  cfblk7 : Squeeze
  cfblk8 : Rounding
  cfblk9 : simulink/Math Operations/Slider Gain  gain=1  low=0  high=2
  cfblk2 : Outport
  wires:
  cfblk6/1 -> cfblk8/1
  cfblk5/1 -> cfblk12/1(cfblk1)
  cfblk1/1 -> cfblk3/1
  cfblk4/1 -> cfblk11/1(cfblk1)
  cfblk3/1 -> cfblk7/1, cfblk2/1
  cfblk8/1 -> cfblk9/1
  cfblk7/1 -> cfblk10/1(cfblk1)
  cfblk10/1(cfblk2) -> cfblk5/2
  cfblk12/1(cfblk2) -> cfblk13/1
  cfblk13/1 -> cfblk5/1
  cfblk11/1(cfblk2) -> cfblk14/1
  cfblk14/1 -> cfblk4/1
  cfblk9/1 -> cfblk15/1
  cfblk15/1 -> cfblk6/1

== system sampleModel2072_pp/cfblk58 ==
  cfblk1 : Inport
  cfblk10 : Subsystem
  cfblk11 : Subsystem
  cfblk12 : Subsystem
  cfblk13 : Delay  SampleTime=1
  cfblk14 : Delay  SampleTime=1
  cfblk15 : Delay  SampleTime=1
  cfblk3 : pid_lib/PID Controller  Controller=PID  Form=Parallel  TimeDomain=Discrete-time  UseExternalTs=off  SampleTime=1  IntegratorMethod=Forward Euler  FilterMethod=Forward Euler  ControllerParametersSource=internal  P=1  I=1  D=0  UseFilter=on  N=100  TunerSelectOption=Transfer Function Based (PID Tuner App)  InitialConditionSource=internal  InitialConditionForIntegrator=0  InitialConditionForFilter=0  DifferentiatorICPrevScaledInput=0  ExternalReset=none  TrackingMode=off  Kt=1  LimitOutput=off  SatLimitsSource=internal  UpperSaturationLimit=inf  LowerSaturationLimit=-inf  LinearizeAsGain=off  AntiWindupMode=none  Kb=1  POutMin=[]  POutMax=[]  IOutMin=[]  IOutMax=[]  DOutMin=[]  DOutMax=[]  NOutMin=[]  NOutMax=[]  SumOutMin=[]  SumOutMax=[]  SaturationOutMin=[]  SaturationOutMax=[]  PParamMin=[]  PParamMax=[]  IParamMin=[]  IParamMax=[]  DParamMin=[]  DParamMax=[]  NParamMin=[]  NParamMax=[]  KbParamMin=[]  KbParamMax=[]  KtParamMin=[]  KtParamMax=[]  KbOutMin=[]  KbOutMax=[]  KtOutMin=[]  KtOutMax=[]  IntegratorOutMin=[]  IntegratorOutMax=[]  FilterOutMin=[]  FilterOutMax=[]  SumI1OutMin=[]  SumI1OutMax=[]  SumI2OutMin=[]  SumI2OutMax=[]  SumI3OutMin=[]  SumI3OutMax=[]  SumI4OutMin=[]  SumI4OutMax=[]  SumDOutMin=[]  SumDOutMax=[]  DifferentiatorOutMin=[]  DifferentiatorOutMax=[]  FilterDiffOutCoefMin=[]  FilterDiffOutCoefMax=[]  ReciprocalOutMin=[]  ReciprocalOutMax=[]  SumDenOutMin=[]  SumDenOutMax=[]  SumNumOutMin=[]  SumNumOutMax=[]  DivideOutMin=[]  DivideOutMax=[]  UdiffTsProdOutMin=[]  UdiffTsProdOutMax=[]  NTsProdOutMin=[]  NTsProdOutMax=[]  UintegralTsProdOutMin=[]  UintegralTsProdOutMax=[]  UngainTsProdOutMin=[]  UngainTsProdOutMax=[]  IntegratorContinuousStateAttributes=''  IntegratorStateMustResolveToSignalObject=off  IntegratorRTWStateStorageClass=Auto  FilterContinuousStateAttributes=''  FilterStateMustResolveToSignalObject=off  FilterRTWStateStorageClass=Auto  ParallelPVariant=InternalParameters  IdealPVariant=Disabled  IVariant=InternalParameters  DVariant=InternalParameters  IntegratorVariant=Discrete  SatVariant=Disabled  AWVariant=Passthrough  PCopyVariant=Disabled  TRVariant=Disabled  FdbkBlocksVariant=Forward  IdealPFdbkVariant=Disabled  SatFdbkVariant=Disabled  DerivativeFilterVariant=ForwardEulerFilter  NVariant=InternalParameters  NCopyVariant=Disabled  FilterICVariant=InternalICsFilter  IntegratorICVariant=InternalICs  ExternalResetVariant=Disabled  TRSumVariant=Passthrough  SumFdbkVariant=Disabled  SumVariant=Sum_PID  TsampFilterVariant=InternalTs  TsampNgainVariant=Passthrough  TsampIntegralVariant=Passthrough  ExternalSaturationOutDataTypeStr=Inherit: Same as second input
  cfblk4 : Product  Inputs=*
  cfblk5 : simulink/Math Operations/MinMax Running Resettable  Function=min  vinit=0.0
  cfblk6 : Gain  Gain=[-79769264.902047]
  cfblk7 : Subsystem
  cfblk8 : Subsystem
  cfblk9 : Subsystem
  cfblk2 : Outport
  wires:
  cfblk10/1(cfblk2) -> cfblk6/1
  cfblk10/2(cfblk14) -> cfblk12/1(cfblk1)
  cfblk4/1 -> cfblk8/1(cfblk1)
  cfblk1/1 -> cfblk10/1(cfblk1), cfblk2/1
  cfblk6/1 -> cfblk12/2(cfblk13)
  cfblk12/1(cfblk2) -> cfblk9/1(cfblk1)
  cfblk3/1 -> cfblk5/1
  cfblk5/1 -> cfblk4/1
  cfblk11/1(cfblk2) -> cfblk3/1, cfblk15/1
  cfblk7/1(cfblk2) -> cfblk11/1(cfblk1)
  cfblk9/1(cfblk2) -> cfblk13/1
  cfblk13/1 -> cfblk10/2(cfblk13)
  cfblk8/1(cfblk2) -> cfblk14/1
  cfblk14/1 -> cfblk5/2
  cfblk15/1 -> cfblk7/1(cfblk1)

== system sampleModel2072_pp/cfblk59 ==
  cfblk1 : Inport
  cfblk10 : Math  Operator=log  SaturateOnIntegerOverflow=on
  cfblk11 : simulink/Math Operations/Slider Gain  gain=1  low=0  high=2
  cfblk12 : Subsystem
  cfblk13 : Subsystem
  cfblk14 : Delay  SampleTime=1
  cfblk15 : Delay  SampleTime=1
  cfblk3 : Delay  SampleTime=1
  cfblk4 : Delay  DelayLengthSource=Input port  SampleTime=1
      settings: InputPortMap=u0,p1
  cfblk5 : Sqrt  SaturateOnIntegerOverflow=on
  cfblk6 : Abs
  cfblk7 : Sum  Inputs=+-
  cfblk8 : Bias  Bias=[-273154549.784259]
  cfblk9 : Product
  cfblk2 : Outport
  wires:
  cfblk7/1 -> cfblk3/1
  cfblk3/1 -> cfblk11/1
  cfblk13/1(cfblk2) -> cfblk12/1(cfblk1)
  cfblk9/1 -> cfblk2/1
  cfblk6/1 -> cfblk13/1(cfblk1), cfblk7/2
  cfblk8/1 -> cfblk9/1
  cfblk4/1 -> cfblk5/1
  cfblk11/1 -> cfblk8/1
  cfblk5/1 -> cfblk6/1, cfblk15/1
  cfblk1/1 -> cfblk9/2
  cfblk12/1(cfblk2) -> cfblk7/1, cfblk10/1
  cfblk10/1 -> cfblk14/1
  cfblk14/1 -> cfblk4/1
  cfblk15/1 -> cfblk4/2

== system sampleModel2072_pp/cfblk60 ==
  cfblk1 : Inport
  cfblk8 : Inport  Port=2
  cfblk3 : pid_lib/PID Controller  Controller=PID  Form=Parallel  TimeDomain=Discrete-time  UseExternalTs=off  SampleTime=1  IntegratorMethod=Forward Euler  FilterMethod=Forward Euler  ControllerParametersSource=internal  P=1  I=1  D=0  UseFilter=on  N=100  TunerSelectOption=Transfer Function Based (PID Tuner App)  InitialConditionSource=internal  InitialConditionForIntegrator=0  InitialConditionForFilter=0  DifferentiatorICPrevScaledInput=0  ExternalReset=none  TrackingMode=off  Kt=1  LimitOutput=off  SatLimitsSource=internal  UpperSaturationLimit=inf  LowerSaturationLimit=-inf  LinearizeAsGain=off  AntiWindupMode=none  Kb=1  POutMin=[]  POutMax=[]  IOutMin=[]  IOutMax=[]  DOutMin=[]  DOutMax=[]  NOutMin=[]  NOutMax=[]  SumOutMin=[]  SumOutMax=[]  SaturationOutMin=[]  SaturationOutMax=[]  PParamMin=[]  PParamMax=[]  IParamMin=[]  IParamMax=[]  DParamMin=[]  DParamMax=[]  NParamMin=[]  NParamMax=[]  KbParamMin=[]  KbParamMax=[]  KtParamMin=[]  KtParamMax=[]  KbOutMin=[]  KbOutMax=[]  KtOutMin=[]  KtOutMax=[]  IntegratorOutMin=[]  IntegratorOutMax=[]  FilterOutMin=[]  FilterOutMax=[]  SumI1OutMin=[]  SumI1OutMax=[]  SumI2OutMin=[]  SumI2OutMax=[]  SumI3OutMin=[]  SumI3OutMax=[]  SumI4OutMin=[]  SumI4OutMax=[]  SumDOutMin=[]  SumDOutMax=[]  DifferentiatorOutMin=[]  DifferentiatorOutMax=[]  FilterDiffOutCoefMin=[]  FilterDiffOutCoefMax=[]  ReciprocalOutMin=[]  ReciprocalOutMax=[]  SumDenOutMin=[]  SumDenOutMax=[]  SumNumOutMin=[]  SumNumOutMax=[]  DivideOutMin=[]  DivideOutMax=[]  UdiffTsProdOutMin=[]  UdiffTsProdOutMax=[]  NTsProdOutMin=[]  NTsProdOutMax=[]  UintegralTsProdOutMin=[]  UintegralTsProdOutMax=[]  UngainTsProdOutMin=[]  UngainTsProdOutMax=[]  IntegratorContinuousStateAttributes=''  IntegratorStateMustResolveToSignalObject=off  IntegratorRTWStateStorageClass=Auto  FilterContinuousStateAttributes=''  FilterStateMustResolveToSignalObject=off  FilterRTWStateStorageClass=Auto  ParallelPVariant=InternalParameters  IdealPVariant=Disabled  IVariant=InternalParameters  DVariant=InternalParameters  IntegratorVariant=Discrete  SatVariant=Disabled  AWVariant=Passthrough  PCopyVariant=Disabled  TRVariant=Disabled  FdbkBlocksVariant=Forward  IdealPFdbkVariant=Disabled  SatFdbkVariant=Disabled  DerivativeFilterVariant=ForwardEulerFilter  NVariant=InternalParameters  NCopyVariant=Disabled  FilterICVariant=InternalICsFilter  IntegratorICVariant=InternalICs  ExternalResetVariant=Disabled  TRSumVariant=Passthrough  SumFdbkVariant=Disabled  SumVariant=Sum_PID  TsampFilterVariant=InternalTs  TsampNgainVariant=Passthrough  TsampIntegralVariant=Passthrough  ExternalSaturationOutDataTypeStr=Inherit: Same as second input
  cfblk4 : MinMax  Function=max
  cfblk5 : Polyval  Coefs=[ +2.081618890e-019, -1.441693666e-014, +4.719686976e-010, -8.536869453e-006, +1.621573104e-001, -8.087801117e+001 ]
  cfblk6 : Subsystem
  cfblk7 : Subsystem
  cfblk2 : Outport
  wires:
  cfblk7/1(cfblk2) -> cfblk2/1
  cfblk3/1 -> cfblk6/1(cfblk1)
  cfblk6/1(cfblk2) -> cfblk5/1
  cfblk4/1 -> cfblk3/1
  cfblk8/1 -> cfblk7/1(cfblk1)
  cfblk1/1 -> cfblk4/1

== system sampleModel2072_pp/cfblk63 ==
  cfblk1 : Inport
  Action Port : ActionPort  ActionPortLabel=if(u1 >= 0)
  cfblk3 : Assignment  DiagnosticForDimensions=Warning  IndexOptions=Index vector (dialog)  Indices=1  OutputSizes=1
  cfblk4 : Sin  TimeSource=Use external signal  SampleTime=0
  cfblk5 : Subsystem
  cfblk6 : Subsystem
  cfblk7 : Subsystem
  cfblk8 : Delay
  cfblk9 : Delay
  cfblk2 : Outport
  wires:
  cfblk7/1(cfblk2) -> cfblk4/1
  cfblk4/1 -> cfblk2/1, cfblk8/1, cfblk9/1
  cfblk5/1(cfblk2) -> cfblk6/1(cfblk1)
  cfblk1/1 -> cfblk3/1
  cfblk3/1 -> cfblk5/1(cfblk1)
  cfblk6/1(cfblk2) -> cfblk7/1(cfblk1)
  cfblk8/1 -> cfblk6/2(cfblk15)
  cfblk9/1 -> cfblk3/2

== system sampleModel2072_pp/cfblk64 ==
  cfblk1 : Inport
  Action Port : ActionPort  ActionPortLabel=else
  cfblk3 : pid_lib/PID Controller  Controller=PID  Form=Parallel  TimeDomain=Discrete-time  UseExternalTs=off  SampleTime=-1  IntegratorMethod=Forward Euler  FilterMethod=Forward Euler  ControllerParametersSource=internal  P=1  I=1  D=0  UseFilter=on  N=100  TunerSelectOption=Transfer Function Based (PID Tuner App)  InitialConditionSource=internal  InitialConditionForIntegrator=0  InitialConditionForFilter=0  DifferentiatorICPrevScaledInput=0  ExternalReset=none  TrackingMode=off  Kt=1  LimitOutput=off  SatLimitsSource=internal  UpperSaturationLimit=inf  LowerSaturationLimit=-inf  LinearizeAsGain=off  AntiWindupMode=none  Kb=1  POutMin=[]  POutMax=[]  IOutMin=[]  IOutMax=[]  DOutMin=[]  DOutMax=[]  NOutMin=[]  NOutMax=[]  SumOutMin=[]  SumOutMax=[]  SaturationOutMin=[]  SaturationOutMax=[]  PParamMin=[]  PParamMax=[]  IParamMin=[]  IParamMax=[]  DParamMin=[]  DParamMax=[]  NParamMin=[]  NParamMax=[]  KbParamMin=[]  KbParamMax=[]  KtParamMin=[]  KtParamMax=[]  KbOutMin=[]  KbOutMax=[]  KtOutMin=[]  KtOutMax=[]  IntegratorOutMin=[]  IntegratorOutMax=[]  FilterOutMin=[]  FilterOutMax=[]  SumI1OutMin=[]  SumI1OutMax=[]  SumI2OutMin=[]  SumI2OutMax=[]  SumI3OutMin=[]  SumI3OutMax=[]  SumI4OutMin=[]  SumI4OutMax=[]  SumDOutMin=[]  SumDOutMax=[]  DifferentiatorOutMin=[]  DifferentiatorOutMax=[]  FilterDiffOutCoefMin=[]  FilterDiffOutCoefMax=[]  ReciprocalOutMin=[]  ReciprocalOutMax=[]  SumDenOutMin=[]  SumDenOutMax=[]  SumNumOutMin=[]  SumNumOutMax=[]  DivideOutMin=[]  DivideOutMax=[]  UdiffTsProdOutMin=[]  UdiffTsProdOutMax=[]  NTsProdOutMin=[]  NTsProdOutMax=[]  UintegralTsProdOutMin=[]  UintegralTsProdOutMax=[]  UngainTsProdOutMin=[]  UngainTsProdOutMax=[]  IntegratorContinuousStateAttributes=''  IntegratorStateMustResolveToSignalObject=off  IntegratorRTWStateStorageClass=Auto  FilterContinuousStateAttributes=''  FilterStateMustResolveToSignalObject=off  FilterRTWStateStorageClass=Auto  ParallelPVariant=InternalParameters  IdealPVariant=Disabled  IVariant=InternalParameters  DVariant=InternalParameters  IntegratorVariant=Discrete  SatVariant=Disabled  AWVariant=Passthrough  PCopyVariant=Disabled  TRVariant=Disabled  FdbkBlocksVariant=Forward  IdealPFdbkVariant=Disabled  SatFdbkVariant=Disabled  DerivativeFilterVariant=ForwardEulerFilter  NVariant=InternalParameters  NCopyVariant=Disabled  FilterICVariant=InternalICsFilter  IntegratorICVariant=InternalICs  ExternalResetVariant=Disabled  TRSumVariant=Passthrough  SumFdbkVariant=Disabled  SumVariant=Sum_PID  TsampFilterVariant=InternalTs  TsampNgainVariant=Passthrough  TsampIntegralVariant=Passthrough  ExternalSaturationOutDataTypeStr=Inherit: Same as second input
  cfblk4 : DiscreteZeroPole  Poles=[0 0.5]  Gain=1  SampleTime=-1
  cfblk5 : Trigonometry
  cfblk6 : Subsystem
  cfblk7 : Subsystem
  cfblk8 : Delay
  cfblk2 : Outport
  wires:
  cfblk6/1(cfblk2) -> cfblk5/1
  cfblk4/1 -> cfblk2/1
  cfblk7/1(cfblk2) -> cfblk6/1(cfblk1)
  cfblk3/1 -> cfblk7/1(cfblk1)
  cfblk1/1 -> cfblk4/1
  cfblk5/1 -> cfblk8/1
  cfblk8/1 -> cfblk3/1
